simulink model "mdaqdemo_testanalog"  (R2014b)
settings: Solver=FixedStepDiscrete  SolverMode=SingleTasking  StartTime=0.0  StopTime=inf  FixedStep=0.001  RelTol=1e-3
libraries: microdaq_lib x2
settings Model: SimulationMode=external  ExtModeTrigDuration=10000  Creator=peselnikmg  LastModifiedBy=peselnikmg
settings DataIOCC: SignalLoggingSaveFormat=ModelDataLogs
settings OptimizationCC: OptimizeModelRefInitCode=on  LifeSpan=1
settings DebuggingCC: UnderspecifiedInitializationDetection=Classic  MergeDetectMultiDrivingBlocksExec=none  StateNameClashWarn=warning
settings HardwareCC: ProdBitPerLong=40  ProdLargestAtomicInteger=Integer  ProdIntDivRoundTo=Zero  ProdEndianess=LittleEndian  ProdHWDeviceType=Texas Instruments->C6000
settings RTWCC: SystemTargetFile=microdaq.tlc  TemplateMakefile=microdaq.tmf  PostCodeGenCommand=microdaq_postcodegen(buildInfo)  Description=MicroDAQ Real-Time Measurement System  GenerateReport=on  ProcessScript=microdaq_make_rtw_hook  IncludeHyperlinkInReport=on
settings CodeAppCC: IgnoreCustomStorageClasses=off
settings STFCustomTargetCC: CodeReplacementLibrary=TI C674x  CombineOutputUpdateFcns=on  ERTCustomFileBanners=on  SupportContinuousTime=off  SupportNonInlinedSFcns=off  MATLABClassNameForMDSCustomization=Simulink.SoftwareTarget.ERTCustomization  GRTInterface=off  SystemTargetFile=microdaq.tlc
settings ERTTargetCC: CodeReplacementLibrary=TI C674x  ParMdlRefBuildCompliant=off  CompOptLevelCompliant=off  ConcurrentExecutionCompliant=off  ERTFirstTimeCompliant=off  ModelStepFunctionPrototypeControlCompliant=off  CPPClassGenCompliant=off  ExtMode=on  ExtModeStaticAlloc=on  ExtModeStaticAllocSize=10485760  ExtModeMexArgs=getpref('microdaq','TargetIP') 1 4344  InlinedParameterPlacement=NonHierarchical  ERTCustomFileTemplate=microdaq_main.tlc

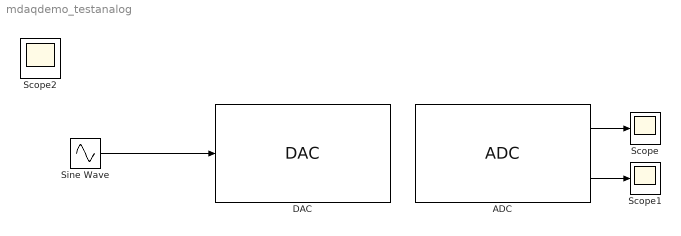
== system mdaqdemo_testanalog ==
  ADC : microdaq_lib/Analog/ADC  Priority=2  pConverter=ADC01 - 8 channel, 166ksps, 12-bit, -/+10V range  pChannel=1  pChannelCount=ones([1 1 ])  pRange=5V  pPolarity=Bipolar  pMode=Single-ended  SampleTime=0.1
      settings: AttributesFormatString=Priority: %<Priority>
  DAC : microdaq_lib/Analog/DAC  Priority=1  pConverter=DAC01 - 8 channel, 12-bit, 0-5V range  pChannel=1  pChannelCount=ones([1 1 ])  pMode=Sequential  pModeTrig=Software  pTermAll=on  pTerm=0.0  SampleTime=0.1
      settings: AttributesFormatString=Priority: %<Priority>
  Scope : Scope
      settings: YMin=0  YMax=16000
  Scope1 : Scope
      settings: YMin=0
  Sine Wave : Sin  Bias=2.5  SampleTime=0.1
      settings: AttributesFormatString=Sample Time: %<SampleTime>
  Scope2 : Scope
      settings: MaxDataPoints=7500
  wires:
  Sine Wave/1 -> DAC/1
  ADC/1 -> Scope/1
  ADC/2 -> Scope1/1
